simulink model "HVDC_VSC_1CPUcore_dcpl"  (Simulink 8.4)
settings: Solver=ode3  SolverMode=SingleTasking  StartTime=0.0  StopTime=70.0  FixedStep=Ts_Power  RelTol=1e-3  AbsTol=1e-2
PreLoadFcn:
  | Ts_Power=50e-6; Ts_Control=1*Ts_Power; init_cosim_IA; startup_transients_hvdc_vsc;
PostLoadFcn:
  | Ts_Power=50e-6; Ts_Control=1*Ts_Power; init_cosim_IA; startup_transients_hvdc_vsc;
InitFcn:
  | Ts_Power=50e-6; Ts_Control=1*Ts_Power; init_cosim_IA; startup_transients_hvdc_vsc;
undefined symbols (not defined in the file): CLARK, D1, Delta, dPref1_2, dPref1_2_rlimit, gcbh, h, intfDelay, level, lib_mesures, magnitude, ResistanceM, rte_drive_private_lib, rte_tsb3level_hiz_rect_cb, sps_rtmsupport, t_deblock_Pref1, t_deblock_Udref2, t_dPref1_2, t_SwitchITMIdc, t_SwitchITMVdc, Ts_intf, TSB3_hiZR
libraries: powerlib x183, spsVIMeasurementModel x102, powerlib_extras x71, powerlib_meascontrol x50, rteventslib x26, op_dpl_lib x20, rtlab x14, sps_avr x6, artemis x1
(part 4 of 13)

== system HVDC_VSC_1CPUcore_dcpl/SS_HVDCStation2_WSCC2/Station 2 (Inverter) ==
  note: Converter Station 2
  note: DC Capacitor
  note: DC Filter
      | 3rd Harmonic
  note: Smoothing reactor
  200 MVA 230:100 kV 0.15 p.u. : powerlib/Elements/Three-Phase Transformer (Two Windings)  Winding1Connection=Yg  UNITS=pu  NominalPower=[200e6 , 60]  Winding1="[230e3 * 1.015   0.0025  0.075]"  Winding2Connection=Delta (D1)  Winding2="[100e3  0.0025  0.075]"  SetSaturation=off  Rm=500  Lm=500  Saturation=[ 0,0 ; 0.012,1.25 ; 1.012,1.6 ]  Hysteresis=off  DataFile='hysteresis'  SetInitialFlux=off  InitialFluxes=[-1.00735070526646 0.511416236666093 0.495934468600514]  Measurements=None  MoreParameters=off  BreakLoop=off  DataType=off  TransfoNumber=0
  A--> pu_AC_sec : Gain  Gain=1/(200e6/100e3/sqrt(3)*sqrt(2))
  Bconv2 : Subsystem  DialogController=POWERSYS.PowerSysDialog  LoadFcn=sps_rtmsupport('LoadFcn',gcbh);  StartFcn=sps_rtmsupport('StartFcn',gcbh);  StopFcn=sps_rtmsupport('StopFcn',gcbh);  mask(Three-Phase VI Measurement){VoltageMeasurement=phase-to-ground, SetLabelV=on, LabelV=Uv_abc2, Vpu=on, VpuLL=off, CurrentMeasurement=yes, SetLabelI=on, LabelI=Iv_abc2, Ipu=on, Pbase=200e6, Vbase=100e3, OutputType=Complex, PhasorSimulation=off, PSBequivalent=0}
      mask prompts: VoltageMeasurement "Voltage measurement"; SetLabelV "Use a label"; LabelV "Signal label  (use a From block to collect this signal)"; Vpu "Voltages in pu,  based on peak value of nominal phase-to-ground voltage"; VpuLL "Voltages in pu,  based on peak value of nominal phase-to-phase  voltage"; CurrentMeasurement "Current measurement"; SetLabelI "Use a label"; LabelI "Signal label  (use a From block to collect this signal)"; Ipu "Currents in pu"; Pbase "Base power ( VA 3 phase)"; Vbase "Nominal voltage used for pu measurement (Vrms phase-phase) :"; OutputType "Output signals in:"; PhasorSimulation "Phasor simulation (internal use)"; PSBequivalent "Equivalent circuit (internal use)"
      mask help:
      | Ideal three-phase voltage and current measurements.
      |
      | The block can output the voltages and currents in per unit values or in volts and amperes.
      mask init: same as HVDC_VSC_1CPUcore_dcpl/SM_WSCC1_HVDCStation1/B1
      settings: CopyFcn=sps_rtmsupport('CopyFcn',gcbh); powericon('ThreePhaseVIMeasurementCopy',gcb)  DeleteFcn=sps_rtmsupport('DeleteFcn',gcbh);  UndoDeleteFcn=sps_rtmsupport('UndoDeleteFcn',gcbh);  ModelCloseFcn=sps_rtmsupport('ModelCloseFcn',gcbh);  PreSaveFcn="sps_rtmsupport('PreSaveFcn',gcbh);  set_param(gcb,'LinkStatus','restore')"  PostSaveFcn=sps_rtmsupport('PostSaveFcn',gcbh);  NameChangeFcn=sps_rtmsupport('NameChangeFcn',gcbh);  PreCopyFcn=sps_rtmsupport('PreCopyFcn',gcbh);  OpenFcn=sps_rtmsupport('OpenFcn',gcbh, [1 2 4 5 6 7 9 -12 13]);  CloseFcn=sps_rtmsupport('CloseFcn',gcbh);  PreDeleteFcn=sps_rtmsupport('PreDeleteFcn',gcbh);
      mask Help: helpview(psbhelp)
      mask TypeOptions VoltageMeasurement: no | phase-to-ground | phase-to-phase
      mask Callback VoltageMeasurement: powericon('ThreePhaseVIMeasurementCback',gcb,'Vselector');
      mask Callback SetLabelV: powericon('ThreePhaseVIMeasurementCback',gcb,'');
      mask Callback Vpu: powericon('ThreePhaseVIMeasurementCback',gcb,'Vpu');
      mask Callback VpuLL: powericon('ThreePhaseVIMeasurementCback',gcb,'VpuLL');
      mask TypeOptions CurrentMeasurement: no | yes
      mask Callback CurrentMeasurement: powericon('ThreePhaseVIMeasurementCback',gcb,'');
      mask Callback SetLabelI: powericon('ThreePhaseVIMeasurementCback',gcb,'');
      mask Callback LabelI: powericon('ThreePhaseVIMeasurementCback',gcb,'');
      mask Callback Ipu: powericon('ThreePhaseVIMeasurementCback',gcb,'');
      mask TypeOptions OutputType: Complex | Real-Imag | Magnitude-Angle | Magnitude
  Bfilter2 : Subsystem  DialogController=POWERSYS.PowerSysDialog  LoadFcn=sps_rtmsupport('LoadFcn',gcbh);  StartFcn=sps_rtmsupport('StartFcn',gcbh);  StopFcn=sps_rtmsupport('StopFcn',gcbh);  mask(Three-Phase VI Measurement){VoltageMeasurement=phase-to-ground, SetLabelV=on, LabelV=Uf_abc2, Vpu=on, VpuLL=off, CurrentMeasurement=no, SetLabelI=off, LabelI=Iabc, Ipu=off, Pbase=100e6, Vbase=100e3, OutputType=Complex, PhasorSimulation=off, PSBequivalent=0}
      mask prompts: VoltageMeasurement "Voltage measurement"; SetLabelV "Use a label"; LabelV "Signal label  (use a From block to collect this signal)"; Vpu "Voltages in pu,  based on peak value of nominal phase-to-ground voltage"; VpuLL "Voltages in pu,  based on peak value of nominal phase-to-phase  voltage"; CurrentMeasurement "Current measurement"; SetLabelI "Use a label"; LabelI "Signal label  (use a From block to collect this signal)"; Ipu "Currents in pu"; Pbase "Base power ( VA 3 phase)"; Vbase "Nominal voltage used for pu measurement (Vrms phase-phase) :"; OutputType "Output signals in:"; PhasorSimulation "Phasor simulation (internal use)"; PSBequivalent "Equivalent circuit (internal use)"
      mask help:
      | Ideal three-phase voltage and current measurements.
      |
      | The block can output the voltages and currents in per unit values or in volts and amperes.
      mask init: same as HVDC_VSC_1CPUcore_dcpl/SM_WSCC1_HVDCStation1/B1
      settings: CopyFcn=sps_rtmsupport('CopyFcn',gcbh); powericon('ThreePhaseVIMeasurementCopy',gcb)  DeleteFcn=sps_rtmsupport('DeleteFcn',gcbh);  UndoDeleteFcn=sps_rtmsupport('UndoDeleteFcn',gcbh);  ModelCloseFcn=sps_rtmsupport('ModelCloseFcn',gcbh);  PreSaveFcn="sps_rtmsupport('PreSaveFcn',gcbh);  set_param(gcb,'LinkStatus','restore')"  PostSaveFcn=sps_rtmsupport('PostSaveFcn',gcbh);  NameChangeFcn=sps_rtmsupport('NameChangeFcn',gcbh);  PreCopyFcn=sps_rtmsupport('PreCopyFcn',gcbh);  OpenFcn=sps_rtmsupport('OpenFcn',gcbh, [1 2 4 5 6 7 9 -12 13]);  CloseFcn=sps_rtmsupport('CloseFcn',gcbh);  PreDeleteFcn=sps_rtmsupport('PreDeleteFcn',gcbh);
      mask Help: helpview(psbhelp)
      mask TypeOptions VoltageMeasurement: no | phase-to-ground | phase-to-phase
      mask Callback VoltageMeasurement: powericon('ThreePhaseVIMeasurementCback',gcb,'Vselector');
      mask Callback SetLabelV: powericon('ThreePhaseVIMeasurementCback',gcb,'');
      mask Callback Vpu: powericon('ThreePhaseVIMeasurementCback',gcb,'Vpu');
      mask Callback VpuLL: powericon('ThreePhaseVIMeasurementCback',gcb,'VpuLL');
      mask TypeOptions CurrentMeasurement: no | yes
      mask Callback CurrentMeasurement: powericon('ThreePhaseVIMeasurementCback',gcb,'');
      mask Callback SetLabelI: powericon('ThreePhaseVIMeasurementCback',gcb,'');
      mask Callback LabelI: powericon('ThreePhaseVIMeasurementCback',gcb,'');
      mask Callback Ipu: powericon('ThreePhaseVIMeasurementCback',gcb,'');
      mask TypeOptions OutputType: Complex | Real-Imag | Magnitude-Angle | Magnitude
  Cn2 : powerlib/Elements/Series RLC Branch  LConnTagsString=__new0  RConnTagsString=__new0  BranchType=C  Resistance=[]  Inductance=[]  SetiL0=off  InitialCurrent=0  Capacitance=70e-6  Setx0=off  InitialVoltage=0  Measurements=None
  Cn_DCF2 : powerlib/Elements/Series RLC Branch  LConnTagsString=__new0  RConnTagsString=__new0  BranchType=C  Resistance=[]  Inductance=[]  SetiL0=off  InitialCurrent=0  Capacitance=12e-6  Setx0=off  InitialVoltage=0  Measurements=None
  Cp2 : powerlib/Elements/Series RLC Branch  LConnTagsString=__new0  RConnTagsString=__new0  BranchType=C  Resistance=[]  Inductance=[]  SetiL0=off  InitialCurrent=0  Capacitance=70e-6  Setx0=off  InitialVoltage=0  Measurements=None
  Cp_DCF2 : powerlib/Elements/Series RLC Branch  LConnTagsString=__new0  RConnTagsString=__new0  BranchType=C  Resistance=[]  Inductance=[]  SetiL0=off  InitialCurrent=0  Capacitance=12e-6  Setx0=off  InitialVoltage=0  Measurements=None
  Current Measurement : powerlib/Measurements/Current Measurement  PhasorSimulation=off  OutputType=Complex  PSBequivalent=0
  Current Measurement1 : powerlib/Measurements/Current Measurement  PhasorSimulation=off  OutputType=Complex  PSBequivalent=0
  Filters 60Hz2 : Subsystem
      mask Display: disp('AC filters\n80 Mvar')
  L_DCF2 : powerlib/Elements/Series RLC Branch  LConnTagsString=__new0  RConnTagsString=__new0  BranchType=RL  Resistance=0.14737  Inductance=46.908e-3  SetiL0=off  InitialCurrent=0  Capacitance=[]  Setx0=off  InitialVoltage=0  Measurements=None
  Ln2 : powerlib/Elements/Series RLC Branch  LConnTagsString=__new0  RConnTagsString=__new0  BranchType=RL  Resistance=0.0251  Inductance=8.0e-3  SetiL0=off  InitialCurrent=0  Capacitance=[]  Setx0=off  InitialVoltage=0  Measurements=Branch current
  Lp2 : powerlib/Elements/Series RLC Branch  LConnTagsString=__new0  RConnTagsString=__new0  BranchType=RL  Resistance=0.0251  Inductance=8.0e-3  SetiL0=off  InitialCurrent=0  Capacitance=[]  Setx0=off  InitialVoltage=0  Measurements=Branch current
  Mux1 : Mux  Inputs=2
  Mux2 : Mux  Inputs=2
  Phase reactor 0.15 p.u. : powerlib/Elements/Three-Phase Series RLC Branch  LConnTagsString=A|B|C  RConnTagsString=A|B|C  BranchType=RL  Resistance=(0.15/100)*(100^2 / 200)  Inductance=0.15 * (100^2 / 200) / (2*pi*50)  Capacitance=1.0  Measurements=None
  TSB3_hiZR1 : Subsystem  AncestorBlock=rte_drive_private_lib/TSB3_hiZR  InitFcn=rte_tsb3level_hiz_rect_cb('InitFcn');  mask(3-Level TSB){legs=3, OutputType=Simulink double (mean model), Ron=0.0001, Vf=0, Ron_dio=0.0001, Vf_dio=0, NbMaxEvents=5, Rhi=2000, Snubber=0, Rsnu=22000, Common_mode_removal=off, dtct=1}
      mask prompts: legs "Number of bridge arms"; OutputType "Voltage output data type"; Ron "Active Switch Ron [ohms]"; Vf "Active Switch Forward voltage Vf [V]"; Ron_dio "Diode Ron [ohms]"; Vf_dio "Diode Forward voltage [V]"; NbMaxEvents "Maximum number of events"; Rhi "Hi impedance value (Ohms)"; Snubber "Emulate snubber effect"; Rsnu "Snubber Resistance Value"; Common_mode_removal "DC link current Common Mode Removal"; dtct "Dead Time current threshold (A)"
      mask help: The RTE-Drive 3-Level TSB block implements a 3-level bridge for which the gates are controlled by RTE signals.
      mask Help: eval('rte_help(''openhelp'',''RTE-Drive 3-Level Tsb'');');
      mask TypeOptions legs: 1 | 2 | 3
      mask TypeOptions OutputType: RT-Events RTE double (high precision model) | Simulink double (mean model) | SimPowerSystem PM (mean model)
      mask Display: plot([0 NaN 105 NaN 78.75 70.35 87.15 78.75 70.35 87.15 78.75 78.75 NaN 52.5 52.5 52.5 78.75 NaN 52.5 52.5 52.5 78.75 78.75 NaN 52.5 52.5 NaN 52.5 52.5 42 NaN 21 31.5 31.5 34.65 31.5 31.5],[0 NaN 111 NaN 59.94 46.62 46.62 59.94 59.94 59.94 59.94 73.26 NaN 99.9 74.37 74.37 74.37 NaN 11.1 33.3 33.3 33.3 46.62 NaN 74.37 63.27 NaN 33.3 44.4 55.5 NaN 49.95 49.95 53.28 49.95 46.62 49.95]);
  V--> pu_AC_sec : Gain  Gain=1/(100e3/sqrt(3)*sqrt(2))
  Voltage Measurement : powerlib/Measurements/Voltage Measurement  PhasorSimulation=off  OutputType=Complex  PSBequivalent=0
  Voltage Measurement1 : powerlib/Measurements/Voltage Measurement  PhasorSimulation=off  OutputType=Complex  PSBequivalent=0
  A : PMIOPort  Port=1  Side=Left
  B : PMIOPort  Port=2  Side=Left
  C : PMIOPort  Port=3  Side=Left
  Pos : PMIOPort  Tag=PMCPort  Port=4  Side=Right
  N : PMIOPort  Tag=PMCPort  Port=5  Side=Right
  Neg : PMIOPort  Tag=PMCPort  Port=6  Side=Right
  tag scope: IdcPN2=global, VdcPN2=global
  wires:
  Mux1/1 -> V--> pu_AC_sec/1
  Voltage Measurement1/1 -> Mux1/2
  Voltage Measurement/1 -> Mux1/1
  Mux2/1 -> A--> pu_AC_sec/1
  Current Measurement1/1 -> Mux2/2
  Current Measurement/1 -> Mux2/1
  A--> pu_AC_sec/1 -> [IdcPN2]
  V--> pu_AC_sec/1 -> [VdcPN2]
  [Pulses2] -> TSB3_hiZR1/1(g)
  connections:
  Bfilter2/RConn1 -- Filters 60Hz2/LConn1 -- Phase reactor 0.15 p.u./LConn1
  Bfilter2/RConn3 -- Filters 60Hz2/LConn3 -- Phase reactor 0.15 p.u./LConn3
  Bfilter2/RConn2 -- Filters 60Hz2/LConn2 -- Phase reactor 0.15 p.u./LConn2
  200 MVA 230:100 kV 0.15 p.u./RConn3 -- Bfilter2/LConn3
  200 MVA 230:100 kV 0.15 p.u./RConn2 -- Bfilter2/LConn2
  200 MVA 230:100 kV 0.15 p.u./RConn1 -- Bfilter2/LConn1
  Current Measurement1/RConn1 -- Neg/RConn1
  Current Measurement/RConn1 -- Pos/RConn1
  TSB3_hiZR1/LConn1 -- Voltage Measurement/LConn1 -- Cp_DCF2/LConn1 -- Lp2/LConn1 -- Cp2/LConn1
  TSB3_hiZR1/LConn3 -- Cn_DCF2/RConn1 -- Ln2/LConn1 -- Voltage Measurement1/LConn1 -- Cn2/RConn1
  TSB3_hiZR1/LConn2 -- Voltage Measurement/LConn2 -- Voltage Measurement1/LConn2 -- Cn2/LConn1 -- L_DCF2/LConn1 -- N/RConn1 -- Cp2/RConn1
  Phase reactor 0.15 p.u./RConn3 -- Bconv2/LConn3
  Phase reactor 0.15 p.u./RConn2 -- Bconv2/LConn2
  Phase reactor 0.15 p.u./RConn1 -- Bconv2/LConn1
  C/RConn1 -- 200 MVA 230:100 kV 0.15 p.u./LConn3
  B/RConn1 -- 200 MVA 230:100 kV 0.15 p.u./LConn2
  A/RConn1 -- 200 MVA 230:100 kV 0.15 p.u./LConn1
  Cn_DCF2/LConn1 -- Cp_DCF2/RConn1 -- L_DCF2/RConn1
  Lp2/RConn1 -- Current Measurement/LConn1
  Ln2/RConn1 -- Current Measurement1/LConn1
  Bconv2/RConn2 -- TSB3_hiZR1/RConn2
  Bconv2/RConn1 -- TSB3_hiZR1/RConn1
  Bconv2/RConn3 -- TSB3_hiZR1/RConn3

== system HVDC_VSC_1CPUcore_dcpl/SS_HVDCStation2_WSCC2/VSC Controller (Station 2) ==
  note: VSC Controller
      | (Station 2)
  note: |----------------Ts_Power--------------|
  note: Sample time:
  note: |------------Ts_Power------------|
  note: |---------------------------Ts_Control-------------------------|
  note: Reference Steps
  note: RTE Firing Pulse unit
  2*pi1 : Gain  Gain=2*pi  SaturateOnIntegerOverflow=on  OutDataTypeStr=Inherit: Same as input  ParamDataTypeStr=Inherit: Same as input
  3-level firing pulse unit for TSB : Subsystem  mask(3-phase RT-Event Discrete PWM Generator){Ts=Ts_Power}
      mask prompts: Ts "Sample time:"
  Anti-aliasing Filters : Subsystem  mask(Anti-aliasing (2nd order lowpass)){f0_aa=2000, Ts=Ts_Power}
      mask prompts: f0_aa "Cut-off frequency (Hz):"; Ts "Sample time:"
      mask init:
      | zeta = 1/sqrt(2);
  Block : Step  Time=t_deblock_Udref2  Before=1  After=0  SampleTime=Ts_Control
  Constant{1..3,5..6} (5 alike) : Constant  Value=0
  Constant4 : Constant  Value=0.0
  Constant7 : Constant  Value=0.0
  Constant8 : Constant  Value=1.0
  Discrete 3-phase PWM Generator : powerlib_extras/Discrete  Control Blocks/Discrete 3-phase PWM Generator  ModulatorType=3-level  ModulatorMode=Un-synchronized  nF=27  Fc=27*60  ModulatingSignals=off  m=0.86  Freq=50  Phase=-50  Ts=Ts_Power
  Discrete VSC Controller (Station 2) : Subsystem  mask(Discrete VSC-Based HVDC Controller){Mode=DC Voltage & Reactive  Power, Xnom=[230e3, 100e3, 200e3, 200e6], XP=[20.0, 1.0, -1.0, 1.43], Xdvco=[3.0, 3.0, 1.05, 0.9], XUdc=[2.0, 40.0 ], XQ=[20.0, 0.5, -0.5], Xvco=[3.0, 3.0, 1.05, 0.94], Xcrc=[1.1,  0.8], Xaccc=[0.6, 6.0,  0.3], enable_dcvbc=on, Xdcvbc=[0.2, 0.03], Ts_Control=Ts_Control}
      mask prompts: Mode "Control Mode:"; Xnom "Nominal Voltages and Power: [ Vpcc(Vrms L-L) , Vconv (Vrms L-L),  Vdc (V L-L), Pnom (VA) ]"; XP "P Regulator [ Ki (1/s), Pmax (pu), Pmin (pu), Ramp (pu/s)]"; Xdvco "P Control: Udc Override [ Kp, Ki (1/s), Udc_max (pu), Udc_min (pu)]"; XUdc "DC Voltage Regulator [ Kp, Ki (1/s)]"; XQ "Q Regulator [ Ki (1/s), Qmax (pu), Qmin (pu)]"; Xvco "Q Control: Uac Override [ Kp, Ki (1/s), U_max (pu), U_min (pu)]"; Xcrc "Current Reference Limits [ lim_d (pu),  lim_q (pu)]"; Xaccc "Inner Current Regulator [ Kp, Ki (1/s), Kf (pu)]"; enable_dcvbc "DC Voltage Balance"; Xdcvbc "DC Voltage Balance Control} [ Kp, Ki (1/s)]"; Ts_Control "Sample Time (s)"
      mask help:
      | This block implements a controller for a VSC (Voltage-Sourced Converter) HVDC using a three-level or Neutral Point Clamped (NPC) converter bridge.
      | The 'Vref_abc' output contains the three modulating signals used by  the carrier-based  Sinusoidal Pulse Width Modulation (SPWM) pulse generator.
      | The output  'm' is a bus signal . Use the Bus Selector block to extract individual signals.
      |
      | See the "VSC-Based Transmission Link " tutorial for a description of the control system.
      mask init: same as HVDC_VSC_1CPUcore_dcpl/SM_WSCC1_HVDCStation1/VSC Controller (Station 1)/Discrete VSC Controller (Station 1)
      mask TypeOptions Mode: Active & Reactive Power | DC Voltage & Reactive  Power
      mask Callback Mode:
      | tempMaskVis=get_param(gcb,'MaskVisibilities');
      | if strcmp(get_param(gcb,'Mode'),'Active & Reactive Power')
      | 	tempMaskVis{2}='on'; tempMaskVis{3}='on'; tempMaskVis{4}='on'; tempMaskVis{5}='on';
      | 	tempMaskVis{6}='on'; tempMaskVis{5}='off'; tempMaskVis{8}='on'; tempMaskVis{9}='on';
      | 	tempMaskVis{10}='on';  tempMaskVis{12}='on';
      | 
      | else
      | 	tempMaskVis{2}='on'; tempMaskVis{3}='off'; tempMaskVis{4}='off'; tempMaskVis{5}='on';
      | 	tempMaskVis{6}='on'; tempMaskVis{7}='on'; tempMaskVis{8}='on'; tempMaskVis{9}='on';
      | 	tempMaskVis{10}='on';  tempMaskVis{12}='on';
      | end
      | if strcmp(get_param(gcb,'enable_dcvbc'),'on')
      | 	tempMaskVis{11}='on';
      | else
      | 	tempMaskVis{11}='off';
      | end
      | set_param(gcb,'MaskVisibilities',tempMaskVis);
      mask Callback enable_dcvbc:
      | tempMaskVis=get_param(gcb,'MaskVisibilities');
      | if strcmp(get_param(gcb,'enable_dcvbc'),'on')
      | 	tempMaskVis{11}='on';
      | else
      | 	tempMaskVis{11}='off';
      | end
      | set_param(gcb,'MaskVisibilities',tempMaskVis);
  Discrete-Time Integrator2 : DiscreteIntegrator  SampleTime=Ts_Power
  Sum3 : Sum  SaturateOnIntegerOverflow=on
  Switch : Switch  Threshold=0.5  SaturateOnIntegerOverflow=on
  Switch1 : Switch  Threshold=0.5  SaturateOnIntegerOverflow=on
  Switch2 : Switch  Threshold=0.5  SaturateOnIntegerOverflow=on
  Switching_Frequency : Constant  Value=27*60
  Terminator : Terminator
  Unit Delay : UnitDelay  SampleTime=Ts_Control
  tag scope: Control2=global, Pulses2=global, Qref2=global, Udref2=global, Vref_abc2=global
  wires:
  Block/1 -> Switch/2, Discrete VSC Controller (Station 2)/11(block_status), Switch1/2
  Discrete 3-phase PWM Generator/1 -> Switch/3
  Constant2/1 -> Switch/1
  Unit Delay/1 -> Discrete 3-phase PWM Generator/1, 3-level firing pulse unit for TSB/1(3 phase output frequency)
  [Iv_abc2] -> Anti-aliasing Filters/4("Iv_abc ")
  [Uf_abc2] -> Anti-aliasing Filters/3("Uf_abc  ")
  [Iabc_B2] -> Anti-aliasing Filters/2("Iabc ")
  [Uabc_B2] -> Anti-aliasing Filters/1("Uabc ")
  Discrete 3-phase PWM Generator/2 -> Terminator/1
  [VdcPN2] -> Anti-aliasing Filters/5("Udc_pn  ")
  [IdcPN2] -> Anti-aliasing Filters/6("Idc_pn ")
  Anti-aliasing Filters/1(Uabc) -> Discrete VSC Controller (Station 2)/1(Uabc (pu))
  Anti-aliasing Filters/2(Iabc) -> Discrete VSC Controller (Station 2)/2(Iabc (pu))
  Anti-aliasing Filters/3(Uf_abc) -> Discrete VSC Controller (Station 2)/3(Uf_abc (pu))
  Anti-aliasing Filters/4(" Iv_abc") -> Discrete VSC Controller (Station 2)/4(Iv_abc (pu))
  Anti-aliasing Filters/5("Udc_pn ") -> Discrete VSC Controller (Station 2)/5(Udc_pn (pu))
  Anti-aliasing Filters/6(" Idc_pn") -> Discrete VSC Controller (Station 2)/6(Idc_pn (pu))
  Constant3/1 -> Discrete VSC Controller (Station 2)/7(Pref)
  Constant8/1 -> [Udref2], Discrete VSC Controller (Station 2)/10(Udref)
  Constant1/1 -> Discrete VSC Controller (Station 2)/8(dPref)
  Discrete VSC Controller (Station 2)/2(m) -> [Control2]
  Discrete VSC Controller (Station 2)/1(Vref_abc) -> Unit Delay/1, [Vref_abc2]
  3-level firing pulse unit for TSB/1(duty) -> Switch1/3
  Constant5/1 -> Switch1/1
  Discrete-Time Integrator2/1 -> 3-level firing pulse unit for TSB/2(wt)
  2*pi1/1 -> Discrete-Time Integrator2/1
  Switching_Frequency/1 -> 2*pi1/1
  Switch1/1 -> Switch2/3
  Switch/1 -> Switch2/1
  Switch2/1 -> [Pulses2]
  Constant6/1 -> Switch2/2
  Constant4/1 -> Sum3/1
  Sum3/1 -> [Qref2], Discrete VSC Controller (Station 2)/9(Qref)
  Constant7/1 -> Sum3/2
